simulink model "MiniTracker_Model"  (R2023b)
settings: Solver=VariableStepAuto  StartTime=0.0  StopTime=100  RelTol=1e-3
undefined symbols (not defined in the file or in its folder): control_net, sensor_model
settings Model: Creator=fikre  LastModifiedBy=fikre

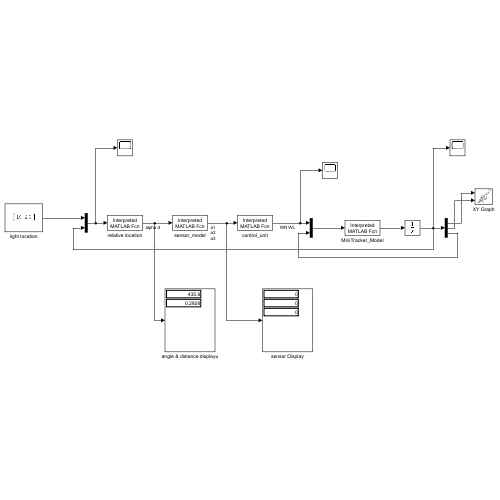
[thumbnail: Simulink's stored preview of the top-level diagram]
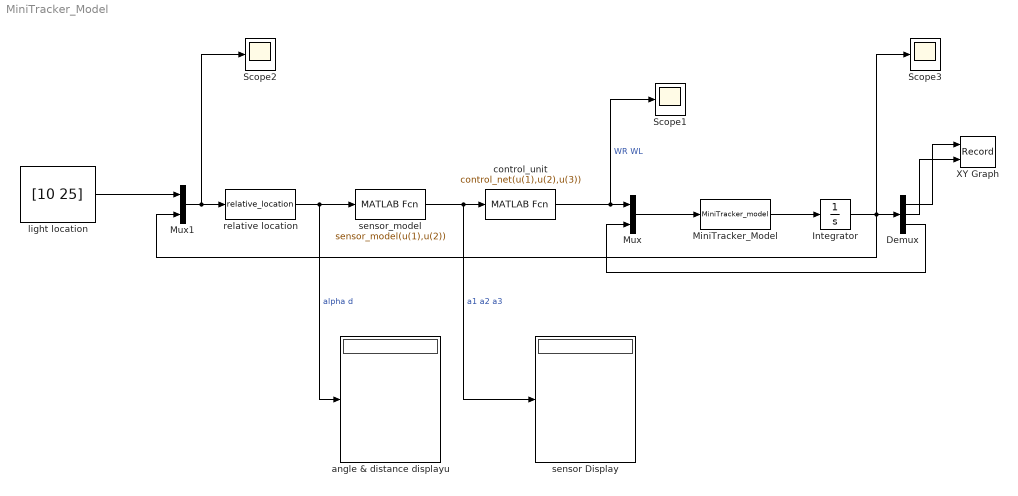
== system MiniTracker_Model ==
  Demux : Demux  Outputs=3
  Integrator : Integrator  InitialCondition=[0 0 pi/2]
  MiniTracker_Model : MATLABFcn  MATLABFcn=MiniTracker_model
  Mux : Mux  Inputs=2
  Mux1 : Mux  Inputs=2
  Scope1 : Scope
  Scope2 : Scope
  Scope3 : Scope
  XY Graph : Record  FileSettingsInternal="{\"entries\":[{\"content\":{\"excelSettings\":{\"content\":{},\"type\":\"Streamout.ExcelSettings\"}},\"type\":\"Streamout.FileSettingStorage\",\"uuid\":\"\"}],\"packageUris\":[\"http:\\/\\/schema.mathworks.com\\/mf0\\/streamout_blocks\\/R2020a\"],\"version\":\"1.0\"}"  Layout=[1 1]  SignalsInternal="{\"entries\":[{\"content\":{\"signals\":[{\"content\":{\"blockPath\":[],\"dimensions\":[1],\"domain\":\"\",\"lineColor\":\"#a2142f\",\"plots\":[ 1 ],\"port\":1,\"sid\":[\"\"],\"signalID\":1,\"signalName\":\"Demux:1\"},\"type\":\"RecordBlkView.Signal\",\"uuid\":\"\"},{\"content\":{\"blockPath\":[],\"dimensions\":[1],\"domain\":\"\",\"lineColor\":\"#139fff\",\"plots\":[ 1 ],\"port\":2,\"sid\":[\"\"],\"signalID\":2,\"signalName\":\"Demux:2\"},\"type\":\"RecordBlkView.Signal\",\"uuid\":\"\"}]},\"type\":\"RecordBlkView.InputSignals\",\"uuid\":\"\"}],\"packageUris\":[\"http:\\/\\/schema.mathworks.com\\/mf0\\/streamout_blocks\\/R2020a\"],\"version\":\"1.0\"}"  VisualizationBindings="{\"xyplotplugin\":{\"info\":[{\"series\":[{\"bindingParametersList\":[{\"parameter\":\"X-Axis\",\"signalID\":1,\"signalName\":\"Demux:1\"},{\"parameter\":\"Y-Axis\",\"signalID\":2,\"signalName\":\"Demux:2\"}],\"seriesID\":0}],\"subplotID\":1}]}}"  CompatibilityTag=XY
  angle & distance displayu : Display
  control_unit : MATLABFcn  MATLABFcn=control_net(u(1),u(2),u(3))
  light location : Constant  Value=[10 25]
  relative location : MATLABFcn  MATLABFcn=relative_location
  sensor Display : Display
  sensor_model : MATLABFcn  MATLABFcn=sensor_model(u(1),u(2))
  wires:
  MiniTracker_Model/1 -> Integrator/1
  Mux/1 -> MiniTracker_Model/1
  Demux/3 -> Mux/2
  control_unit/1 -> Scope1/1, Mux/1  "WR WL"
  Integrator/1 -> Scope3/1, Mux1/2, Demux/1
  Demux/1 -> XY Graph/1
  Demux/2 -> XY Graph/2
  sensor_model/1 -> sensor Display/1, control_unit/1  "a1 a2 a3"
  relative location/1 -> angle & distance displayu/1, sensor_model/1  "alpha d"
  Mux1/1 -> Scope2/1, relative location/1
  light location/1 -> Mux1/1
